simulink model "test"  (R2017b)
settings: Solver=VariableStepAuto  StartTime=0.0  StopTime=10.0  RelTol=1e-3
libraries: simulink x2
settings Model: Creator=Administrator  LastModifiedBy=Administrator

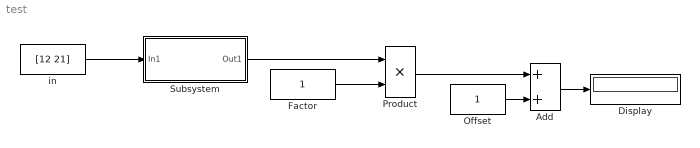
== system test ==
  Add : Sum
  Display : Display
  Factor : Constant
  Offset : Constant
  Product : Product
  Subsystem : Subsystem
  in : Constant  Value=[12 21]
  wires:
  Subsystem/1(Out1) -> Product/1
  Product/1 -> Add/1
  Offset/1 -> Add/2
  Factor/1 -> Product/2
  Add/1 -> Display/1
  in/1 -> Subsystem/1(In1)

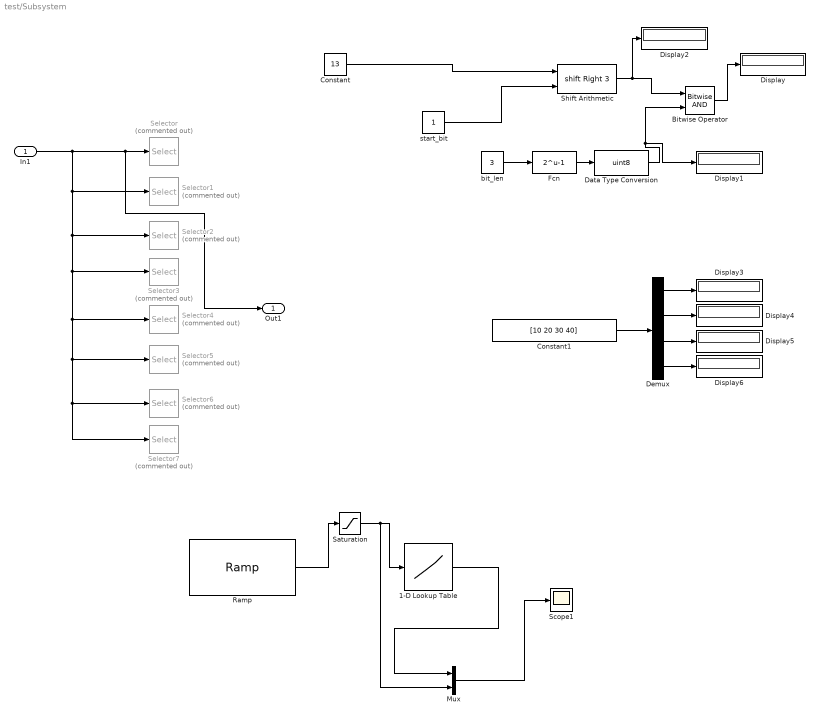
== system test/Subsystem ==
  In1 : Inport
  1-D Lookup Table : Lookup_n-D  NumberOfTableDimensions=1  BreakpointsForDimension1=[-5:5]  Table=tanh([-5:5])  InternalRulePriority=Speed  RndMeth=Simplest  InputSameDT=on
  Bitwise Operator : simulink/Logic and Bit Operations/Bitwise Operator  logicop=AND  UseBitMask=off  NumInputPorts=2  BitMask=bin2dec('11011001')  BitMaskRealWorld=Stored Integer
  Constant : Constant  Value=13  OutDataTypeStr=uint8
  Constant1 : Constant  Value=[10 20 30 40]
  Data Type Conversion : DataTypeConversion  OutDataTypeStr=uint8
  Demux : Demux
  Display{,1..6} (7 alike) : Display
  Fcn : Fcn  Expr=2^u-1
  Mux : Mux  Inputs=2
  Ramp : simulink/Sources/Ramp  slope=5  start=0  X0=-5
  Saturation : Saturate  UpperLimit=5  LowerLimit=-5
  Scope1 : Scope
  Selector : Selector  Commented=on  InputPortWidth=2  IndexOptions=Index vector (dialog)  Indices=[1]  OutputSizes=1
  Selector{1..3,5..7} (6 alike) : Selector  Commented=on  InputPortWidth=2  IndexOptions=Index vector (dialog)  Indices=[2]  OutputSizes=1
  Selector4 : Selector  Commented=on  InputPortWidth=2  IndexOptions=Index vector (dialog)  Indices=[1]  OutputSizes=1
  Shift Arithmetic : ArithShift  BitShiftNumberSource=Input port  BitShiftNumber=3  BitShiftDirection=Right
      settings: InputPortMap=u0,p1
  bit_len : Constant  Value=3
  start_bit : Constant  OutDataTypeStr=uint8
  Out1 : Outport
  wires:
  In1/1 -> Selector1/1, Selector2/1, Selector3/1, Selector4/1, Selector5/1, Selector6/1, Selector7/1, Out1/1, Selector/1
  bit_len/1 -> Fcn/1
  Constant/1 -> Shift Arithmetic/1
  start_bit/1 -> Shift Arithmetic/2
  Data Type Conversion/1 -> Bitwise Operator/2, Display1/1
  Bitwise Operator/1 -> Display/1
  Shift Arithmetic/1 -> Bitwise Operator/1, Display2/1
  Fcn/1 -> Data Type Conversion/1
  Constant1/1 -> Demux/1
  Demux/2 -> Display4/1
  Demux/1 -> Display3/1
  Demux/3 -> Display5/1
  Demux/4 -> Display6/1
  Ramp/1 -> Saturation/1
  1-D Lookup Table/1 -> Mux/1
  Mux/1 -> Scope1/1
  Saturation/1 -> Mux/2, 1-D Lookup Table/1
